simulink model "P8"  (R2020a)
settings: Solver=VariableStepAuto  StartTime=0.0  StopTime=2  RelTol=1e-3
values from neighbouring files (symbols this model uses):
  C = [0, 0, 1]    [P8_SergioPons_v2.m]
  K = place(zA,zB,p)    [P8_SergioPons_v2.m]
  k3 = K(3)    [P8_SergioPons_v2.m]
undefined symbols (not defined in the file or in its folder): zA, zB
settings Model: Creator=Usuario  LastModifiedBy=Usuario

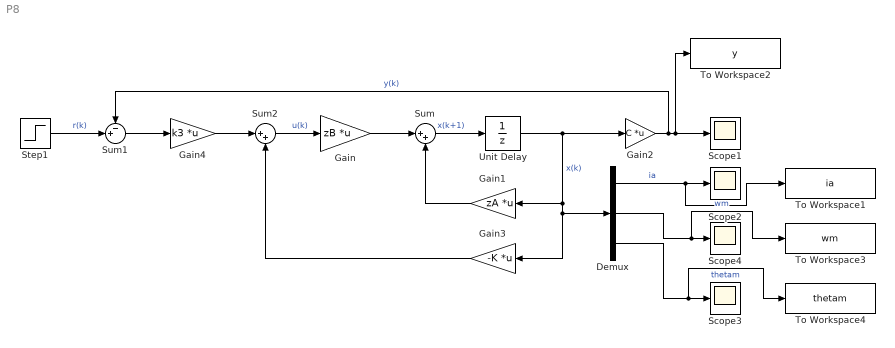
== system P8 ==
  Demux : Demux  Outputs=3
  Gain : Gain  Gain=zB  Multiplication=Matrix(K*u)
  Gain1 : Gain  Gain=zA  Multiplication=Matrix(K*u)
  Gain2 : Gain  Gain=C  Multiplication=Matrix(K*u)
  Gain3 : Gain  Gain=-K  Multiplication=Matrix(K*u)
  Gain4 : Gain  Gain=k3  Multiplication=Matrix(K*u)
  Scope{1..4} (4 alike) : Scope
  Step1 : Step  Time=0  SampleTime=0
  Sum : Sum  Inputs=|++
  Sum1 : Sum  Inputs=-+|
  Sum2 : Sum  Inputs=|++
  To Workspace1 : ToWorkspace  VariableName=ia  SaveFormat=Timeseries  SampleTime=-1
  To Workspace2 : ToWorkspace  VariableName=y  SaveFormat=Timeseries  SampleTime=-1
  To Workspace3 : ToWorkspace  VariableName=wm  SaveFormat=Timeseries  SampleTime=-1
  To Workspace4 : ToWorkspace  VariableName=thetam  SaveFormat=Timeseries  SampleTime=-1
  Unit Delay : UnitDelay  SampleTime=-1  HasFrameUpgradeWarning=on
  wires:
  Sum/1 -> Unit Delay/1  "x(k+1)"
  Unit Delay/1 -> Gain3/1, Demux/1, Gain1/1, Gain2/1  "x(k)"
  Gain2/1 -> Sum1/1, To Workspace2/1, Scope1/1  "y(k)"
  Demux/1 -> To Workspace1/1, Scope2/1  "ia"
  Gain1/1 -> Sum/2
  Demux/2 -> To Workspace3/1, Scope4/1  "wm"
  Demux/3 -> To Workspace4/1, Scope3/1  "thetam"
  Gain/1 -> Sum/1
  Sum1/1 -> Gain4/1
  Gain4/1 -> Sum2/1
  Sum2/1 -> Gain/1  "u(k)"
  Gain3/1 -> Sum2/2
  Step1/1 -> Sum1/2  "r(k)"
